simulink model "fgg"  (R2022b)
settings: Solver=VariableStepAuto  StartTime=0.0  StopTime=10.0  RelTol=1e-3
settings Model: Creator=Asus  LastModifiedBy=Asus

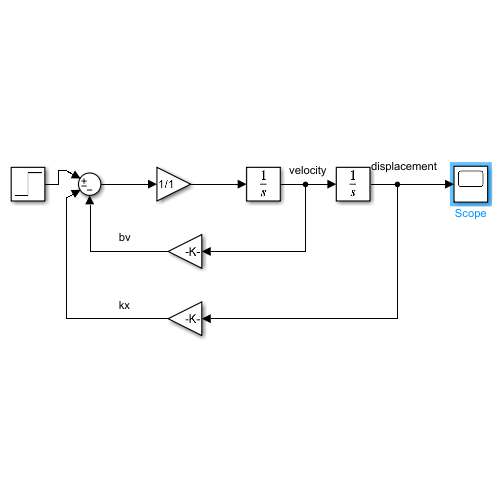
[thumbnail: Simulink's stored preview of the top-level diagram]
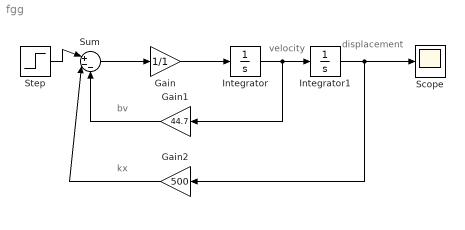
== system fgg ==
  note: displacement
  note: velocity
  note: bv
  note: kx
  Gain : Gain  Gain=1/1
  Gain1 : Gain  Gain=44.7
  Gain2 : Gain  Gain=500
  Integrator : Integrator
  Integrator1 : Integrator
  Scope : Scope
  Step : Step  Time=0  SampleTime=0
  Sum : Sum  Inputs=|+--
  wires:
  Integrator1/1 -> Gain2/1, Scope/1
  Step/1 -> Sum/1
  Sum/1 -> Gain/1
  Gain/1 -> Integrator/1
  Integrator/1 -> Gain1/1, Integrator1/1
  Gain2/1 -> Sum/2
  Gain1/1 -> Sum/3
